simulink library "pitchKp"  (R2022a)
settings: Solver=VariableStepAuto  StartTime=0.0  StopTime=10.0  RelTol=1e-3
undefined symbols (not defined in the file or in its folder): pIp, pitchSP, pKp
libraries: filteredPIDController_ul x1
settings Model: Creator=jcreed2  LastModifiedBy=lhill8
settings SolverCC: AlgebraicLoopSolver=TrustRegion
settings DebuggingCC: UnconnectedInputMsg=warning  UnconnectedOutputMsg=warning  UnconnectedLineMsg=warning  SFMachineParentedDataDiag=warning

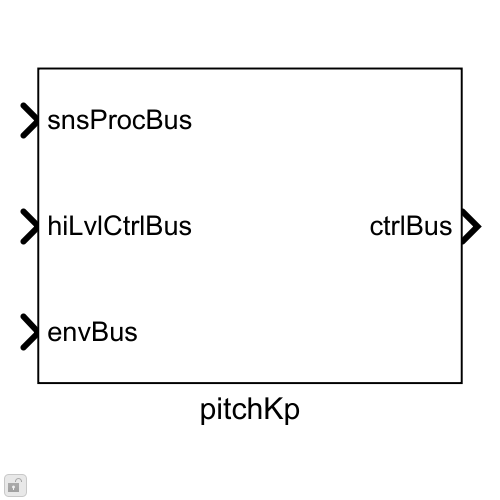
[thumbnail: Simulink's stored preview of the top-level diagram]
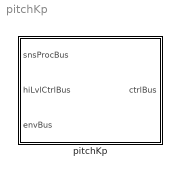
== system pitchKp ==
  pitchKp : Subsystem

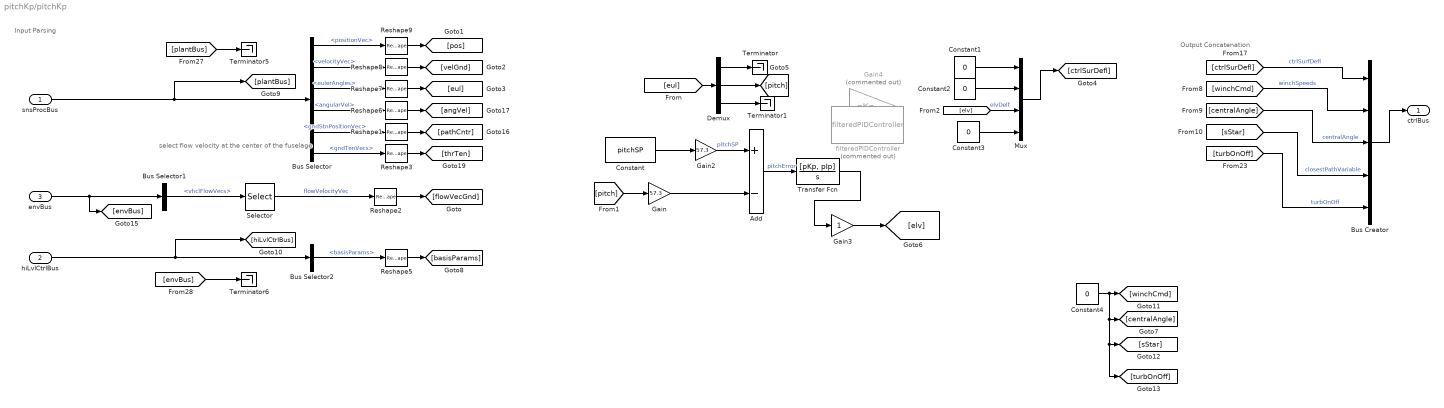
== system pitchKp/pitchKp ==
  note: select flow velocity at the center of the fuselage
  note: Input Parsing
  note: Output Concatenation
  snsProcBus : Inport  OutDataTypeStr=Bus: sensorsProcessingBus
  hiLvlCtrlBus : Inport  Port=2  OutDataTypeStr=Bus: hiLvlCtrlBus
  envBus : Inport  Port=3  OutDataTypeStr=Bus: envBus
  Add : Sum  Inputs=+-
  Bus Creator : BusCreator  Inputs=5  OutDataTypeStr=Bus: fltCtrlBus
      settings: InheritFromInputs=off
  Bus Selector : BusSelector  OutputSignals=positionVec,velocityVec,eulerAngles,angularVel,gndStnPositionVec,gndTenVecs
  Bus Selector1 : BusSelector  OutputSignals=vhclFlowVecs
  Bus Selector2 : BusSelector  OutputSignals=basisParams
  Constant : Constant  Value=pitchSP
  Constant{1..4} (4 alike) : Constant  Value=0
  Demux : Demux  Outputs=3
  Gain : Gain  Gain=57.3
  Gain2 : Gain  Gain=57.3
  Gain3 : Gain
  Gain4 : Gain  Commented=on  Gain=pKp
  Mux : Mux
  Reshape{1..3,5..9} (8 alike) : Reshape  OutputDimensionality=Column vector (2-D)
  Selector : Selector  NumberOfDimensions=2  InputPortWidth=3  IndexOptions=Select all,Index vector (dialog)  Indices=[1 3],5  OutputSizes=1,1
  Terminator{,1,5..6} (4 alike) : Terminator
  Transfer Fcn : TransferFcn  Numerator=[pKp, pIp]  Denominator=[1 0]
  filteredPIDController : filteredPIDController_ul/filteredPIDController  Commented=on  kp=pKp  ki=pIp  kd=0  Value=70  externalReset=none
  ctrlBus : Outport  OutDataTypeStr=Bus: fltCtrlBus  VectorParamsAs1DForOutWhenUnconnected=off
  wires:
  Bus Selector/3 -> Reshape7/1  "<eulerAngles>"
  [envBus] -> Terminator6/1
  Constant4/1 -> [turbOnOff], [sStar], [centralAngle], [winchCmd]
  [pitch] -> Gain/1
  Reshape8/1 -> [velGnd]
  Demux/3 -> Terminator1/1
  Mux/1 -> [ctrlSurDefl]
  [centralAngle] -> Bus Creator/3  "centralAngle"
  Add/1 -> Transfer Fcn/1  "pitchError"
  Bus Selector/6 -> Reshape3/1  "<gndTenVecs>"
  snsProcBus/1 -> Bus Selector/1, [plantBus]
  Selector/1 -> Reshape2/1  "flowVelocityVec"
  Bus Selector2/1 -> Reshape5/1  "<basisParams>"
  Bus Selector/4 -> Reshape6/1  "<angularVel>"
  [eul] -> Demux/1
  Reshape2/1 -> [flowVecGnd]
  Bus Selector1/1 -> Selector/1  "<vhclFlowVecs>"
  envBus/1 -> [envBus], Bus Selector1/1
  hiLvlCtrlBus/1 -> [hiLvlCtrlBus], Bus Selector2/1
  [plantBus] -> Terminator5/1
  [elv] -> Mux/3  "elvDelf"
  Reshape9/1 -> [pos]
  Constant1/1 -> Mux/1
  Reshape6/1 -> [angVel]
  [sStar] -> Bus Creator/4  "closestPathVariable"
  Reshape7/1 -> [eul]
  [winchCmd] -> Bus Creator/2  "winchSpeeds"
  [turbOnOff] -> Bus Creator/5  "turbOnOff"
  [ctrlSurDefl] -> Bus Creator/1  "ctrlSurfDefl"
  Constant3/1 -> Mux/4
  Bus Creator/1 -> ctrlBus/1
  Reshape1/1 -> [pathCntr]
  Reshape5/1 -> [basisParams]
  Reshape3/1 -> [thrTen]
  Bus Selector/1 -> Reshape9/1  "<positionVec>"
  Bus Selector/5 -> Reshape1/1  "<gndStnPositionVec>"
  Bus Selector/2 -> Reshape8/1  "<velocityVec>"
  Constant2/1 -> Mux/2
  Gain3/1 -> [elv]
  Demux/1 -> Terminator/1
  Demux/2 -> [pitch]
  Gain/1 -> Add/2
  Gain2/1 -> Add/1  "pitchSP"
  Constant/1 -> Gain2/1
  Transfer Fcn/1 -> Gain3/1
